simulink model "receiver_overall_reset"  (Simulink 7.5)
settings: Solver=FixedStepDiscrete  SolverMode=SingleTasking  StartTime=0.0  StopTime=(length(simin.signals.values)-1)/Fs  FixedStep=1  RelTol=1e-3
undefined symbols (not defined in the file): Fs
libraries: xbsIndex_r4 x962
(part 3 of 9)

== system receiver_overall_reset/Receiver/Sym-Chooser/7-15 ==
  in : Inport
  clk : Inport  Port=2
  0 : xbsIndex_r4/Constant  arith_type=Unsigned  const=a  n_bits=5  bin_pt=0  explicit_period=off  period=1  equ=P=C  opselect=C  inp2=PCIN>>17  opr=+  inp1=P  carry=CIN  dbl_ovrd=off  block_type=constant
      settings: block_version=12.1
  8 : xbsIndex_r4/Constant  arith_type=Unsigned  const=b  n_bits=5  bin_pt=0  explicit_period=off  period=1  equ=P=C  opselect=C  inp2=PCIN>>17  opr=+  inp1=P  carry=CIN  dbl_ovrd=off  block_type=constant
      settings: block_version=12.1
  Concat : xbsIndex_r4/Concat  num_inputs=2  dbl_ovrd=off  block_type=concat
      settings: block_version=12.1
  Corr0 : Subsystem
  Error0 : xbsIndex_r4/Constant  arith_type=Unsigned  const=16  n_bits=5  bin_pt=0  explicit_period=off  period=1  equ=P=C  opselect=C  inp2=PCIN>>17  opr=+  inp1=P  carry=CIN  dbl_ovrd=off  block_type=constant
      settings: block_version=12.1
  Error1 : xbsIndex_r4/Constant  arith_type=Unsigned  const=16  n_bits=5  bin_pt=0  explicit_period=off  period=1  equ=P=C  opselect=C  inp2=PCIN>>17  opr=+  inp1=P  carry=CIN  dbl_ovrd=off  block_type=constant
      settings: block_version=12.1
  Logical : xbsIndex_r4/Logical  logical_function=XOR  inputs=2  en=on  latency=1  precision=Full  arith_type=Unsigned  n_bits=16  bin_pt=0  align_bp=on  dbl_ovrd=off  block_type=logical
      settings: xl_area=[1 0 0 1 0 0 0]  block_version=12.1
  Mux : xbsIndex_r4/Mux  inputs=4  en=on  latency=1  precision=Full  arith_type=Unsigned  n_bits=16  bin_pt=14  quantization=Truncate  overflow=Wrap  dbl_ovrd=off  block_type=mux
      settings: xl_area=[5 5 0 10 0 0 0]  block_version=12.1
  Negate : xbsIndex_r4/Negate  precision=Full  arith_type="Signed  (2's comp)"  n_bits=16  bin_pt=14  quantization=Truncate  overflow=Wrap  en=off  latency=0  dbl_ovrd=off  block_type=negate
      settings: block_version=12.2
  Relational : xbsIndex_r4/Relational  mode=a>b  en=off  latency=0  dbl_ovrd=off  block_type=relational
      settings: xl_area=[4 1 0 7 0 0 0]  block_version=12.1
  Relational1 : xbsIndex_r4/Relational  mode=a<b  en=off  latency=0  dbl_ovrd=off  block_type=relational
      settings: xl_area=[4 1 0 7 0 0 0]  block_version=12.1
  Thresh : xbsIndex_r4/Constant  arith_type=Unsigned  const=thresh  n_bits=5  bin_pt=0  explicit_period=off  period=1  equ=P=C  opselect=C  inp2=PCIN>>17  opr=+  inp1=P  carry=CIN  dbl_ovrd=off  block_type=constant
      settings: block_version=12.1
  fnd : Outport
  value : Outport  Port=2
  wires:
  Corr0/1(Out1) -> Relational/1, Relational1/1
  Thresh/1 -> Relational/2, Negate/1
  in/1 -> Corr0/1(In1)
  Relational/1 -> Logical/1, Concat/1
  Relational1/1 -> Logical/2, Concat/2
  Logical/1 -> fnd/1
  Error0/1 -> Mux/2
  8/1 -> Mux/3
  Concat/1 -> Mux/1
  0/1 -> Mux/4
  Error1/1 -> Mux/5
  Mux/1 -> value/1
  Negate/1 -> Relational1/2
  clk/1 -> Mux/6, Logical/3

== system receiver_overall_reset/Receiver/Sym-Clk/Corr ==
  In : Inport
  AddSub : xbsIndex_r4/AddSub  mode=Subtraction  use_carryin=off  use_carryout=off  en=off  latency=0  precision=Full  arith_type=Unsigned  n_bits=16  bin_pt=14  quantization=Truncate  overflow=Wrap  dbl_ovrd=off  use_behavioral_HDL=off  hw_selection=Fabric  pipelined=off  block_type=addsub
      settings: xl_area=[4 0 0 6 0 0 0]  block_version=12.1
  Constant0 : xbsIndex_r4/Constant  arith_type=Unsigned  const=1618456172  n_bits=31  bin_pt=0  explicit_period=off  period=1/8  equ=P=C  opselect=C  inp2=PCIN>>17  opr=+  inp1=P  carry=CIN  dbl_ovrd=off  block_type=constant
      settings: block_version=12.1
  Constant1 : xbsIndex_r4/Constant  arith_type=Unsigned  const=31  n_bits=5  bin_pt=0  explicit_period=off  period=1/8  equ=P=C  opselect=C  inp2=PCIN>>17  opr=+  inp1=P  carry=CIN  dbl_ovrd=off  block_type=constant
      settings: block_version=12.1
  Delay_Line : Subsystem  mask{bits=31}
      mask prompts: bits "Number of Bits [2-40]"
      mask init:
      | % save_gcb = gcb
      | % nbits=bits+1
      | % old=find_system(save_gcb,...
      | %     'lookUnderMasks', 'all',...
      | %     'RegExp', 'On',...
      | %     'Name', 'DE\d+');
      | % 
      | %     for i=1:length(old)-1
      | %         delete_line(gcb, ['DE' int2str(i) '/1'], ['DE' int2str(i+1) '/1']);
      | %     end
      | %     for i=1:length(old)
      | %         delete_line(gcb, ['DE' int2str(i) '/2'], ['Concat/' int2str(length(old)-i+1)]);
      | %     end
      | %     delete_line(gcb, '1to2/2', ['Concat/', int2str(length(old)+1)]);
      | %     delete_line(gcb, ['DE' int2str(length(old)) '/1'], ['Terminator/1']);
      | %     for i=2:length(old)
      | %         delete_block(old{i});
      | %     end
      | % 
      | % pos = get_param([save_gcb '/DE1'], 'Position');
      | % width = pos(3)-pos(1);
      | % for i=3:nbits,
      | %     add_block([save_gcb '/DE1'],[save_gcb '/DE' int2str(i-1)],'position',[pos(1)+2*(i-2)*width, pos(2), pos(3)+2*(i-2)*width, pos(4)]);
      | %     add_line(save_gcb, ['DE' int2str(i-2) '/1'], ['DE' int2str(i-1) '/1'], 'autorouting', 'on');    
      | % end
      | % 
      | % posT = get_param([save_gcb '/Terminator'], 'Position');
      | % widthT = posT(3)-posT(1);
      | % heightT = posT(4)-posT(2);
      | % set_param([save_gcb '/Terminator'], 'Position', [pos(1)+2*(nbits-1)*width pos(2) pos(1)+2*(nbits-1)*width+widthT pos(2)+heightT]);
      | % 
      | % add_line(save_gcb, ['DE' int2str(nbits-1) '/1'], ['Terminator/1'], 'autorouting', 'on');
      | % 
      | % posC = get_param([save_gcb '/Concat'], 'Position');
      | % set_param([save_gcb '/Concat'], 'Position', [pos(1)+2*(nbits)*width posC(2) pos(1)+2*(nbits+1)*width posC(2)+2*(nbits-1)*width]);
      | % set_param([save_gcb '/Concat'], 'num_inputs', int2str(nbits));
      | % 
      | % add_line(save_gcb, '1to2/2', ['Concat/' int2str(nbits)], 'autorouting', 'on');
      | % for i=1:nbits-1,
      | %    add_line(save_gcb, ['DE' int2str(i) '/2'], ['Concat/' int2str(nbits-i)], 'autorouting', 'on');
      | % end
      mask StyleString: popup(2|3|4|5|6|7|8|9|10|11|12|13|14|15|16|17|18|19|20|21|22|23|24|25|26|27|28|29|30|31|32|33|34|35|36|37|38|39|40)
  Logical : xbsIndex_r4/Logical  logical_function=XNOR  inputs=2  en=off  latency=0  precision=User Defined  arith_type=Unsigned  n_bits=32  bin_pt=0  align_bp=on  dbl_ovrd=off  block_type=logical
      settings: xl_area=[31 0 0 31 0 0 0]  block_version=12.1
  count 1s : Subsystem
  x 2 : xbsIndex_r4/Shift  shift_dir=Left  shift_bits=1  en=off  latency=0  precision=Full  arith_type=Unsigned  n_bits=7  bin_pt=0  quantization=Truncate  overflow=Wrap  dbl_ovrd=off  block_type=shift
      settings: xl_area=[0 0 0 0 0 0 0]  block_version=12.1
  Out : Outport
  wires:
  Constant0/1 -> Logical/2
  Delay_Line/1(Out) -> Logical/1
  Logical/1 -> count 1s/1(in)
  Constant1/1 -> AddSub/2
  count 1s/1(out) -> x 2/1
  x 2/1 -> AddSub/1
  In/1 -> Delay_Line/1(In)
  AddSub/1 -> Out/1

== system receiver_overall_reset/Rule System/16bit Addresses + PANs/Adresses ==
  Dest Add Type : Inport
  Concat Symbols : Inport  Port=2
  Source Add Type : Inport  Port=3
  Source Add Settings : Inport  Port=4
  Dest Add Settings : Inport  Port=5
  1 : xbsIndex_r4/Constant  arith_type=Unsigned  const=2  n_bits=4  bin_pt=0  explicit_period=off  period=1  equ=P=C  opselect=C  inp2=PCIN>>17  opr=+  inp1=P  carry=CIN  dbl_ovrd=off  block_type=constant
      settings: block_version=12.2
  3 : xbsIndex_r4/Constant  arith_type=Unsigned  const=2  n_bits=4  bin_pt=0  explicit_period=off  period=1  equ=P=C  opselect=C  inp2=PCIN>>17  opr=+  inp1=P  carry=CIN  dbl_ovrd=off  block_type=constant
      settings: block_version=12.2
  Constant : xbsIndex_r4/Constant  arith_type=Unsigned  const=0  n_bits=16  bin_pt=0  explicit_period=off  period=1  equ=P=C  opselect=C  inp2=PCIN>>17  opr=+  inp1=P  carry=CIN  dbl_ovrd=off  block_type=constant
      settings: block_version=12.2
  Delay1 : xbsIndex_r4/Delay  en=off  latency=10  dbl_ovrd=off  reg_retiming=off  block_type=delay
      settings: block_version=12.2
  Delay2 : xbsIndex_r4/Delay  en=off  latency=18  dbl_ovrd=off  reg_retiming=off  block_type=delay
      settings: block_version=12.2
  Dest 16 upper Bound : xbsIndex_r4/Constant  arith_type=Unsigned  const=d16u  n_bits=16  bin_pt=0  explicit_period=off  period=1  equ=P=C  opselect=C  inp2=PCIN>>17  opr=+  inp1=P  carry=CIN  dbl_ovrd=off  block_type=constant
      settings: block_version=12.2
  Dest lower Bound : xbsIndex_r4/Constant  arith_type=Unsigned  const=d16l  n_bits=16  bin_pt=0  explicit_period=off  period=1  equ=P=C  opselect=C  inp2=PCIN>>17  opr=+  inp1=P  carry=CIN  dbl_ovrd=off  block_type=constant
      settings: block_version=12.2
  Logical : xbsIndex_r4/Logical  logical_function=AND  inputs=3  en=off  latency=0  precision=Full  arith_type=Unsigned  n_bits=16  bin_pt=0  align_bp=on  dbl_ovrd=off  block_type=logical
      settings: block_version=12.2
  Logical1 : xbsIndex_r4/Logical  logical_function=AND  inputs=3  en=off  latency=0  precision=Full  arith_type=Unsigned  n_bits=16  bin_pt=0  align_bp=on  dbl_ovrd=off  block_type=logical
      settings: block_version=12.2
  Logical2 : xbsIndex_r4/Logical  logical_function=OR  inputs=2  en=off  latency=0  precision=Full  arith_type=Unsigned  n_bits=16  bin_pt=0  align_bp=on  dbl_ovrd=off  block_type=logical
      settings: block_version=12.2
  Logical3 : xbsIndex_r4/Logical  logical_function=OR  inputs=2  en=off  latency=0  precision=Full  arith_type=Unsigned  n_bits=16  bin_pt=0  align_bp=on  dbl_ovrd=off  block_type=logical
      settings: block_version=12.2
  Logical4 : xbsIndex_r4/Logical  logical_function=OR  inputs=2  en=off  latency=0  precision=Full  arith_type=Unsigned  n_bits=16  bin_pt=0  align_bp=on  dbl_ovrd=off  block_type=logical
      settings: block_version=12.2
  Mux : xbsIndex_r4/Mux  inputs=2  en=off  latency=0  precision=Full  arith_type=Unsigned  n_bits=16  bin_pt=14  quantization=Truncate  overflow=Wrap  dbl_ovrd=off  block_type=mux
      settings: block_version=12.2
  Source 16 low Bound : xbsIndex_r4/Constant  arith_type=Unsigned  const=s16l  n_bits=16  bin_pt=0  explicit_period=off  period=1  equ=P=C  opselect=C  inp2=PCIN>>17  opr=+  inp1=P  carry=CIN  dbl_ovrd=off  block_type=constant
      settings: block_version=12.2
  Source 16 upper Bound : xbsIndex_r4/Constant  arith_type=Unsigned  const=s16u  n_bits=16  bin_pt=0  explicit_period=off  period=1  equ=P=C  opselect=C  inp2=PCIN>>17  opr=+  inp1=P  carry=CIN  dbl_ovrd=off  block_type=constant
      settings: block_version=12.2
  is{1..2,4..5} (4 alike) : xbsIndex_r4/Relational  mode=a>b  en=off  latency=0  dbl_ovrd=off  block_type=relational
      settings: block_version=12.2
  is16 : xbsIndex_r4/Relational  mode=a=b  en=off  latency=0  dbl_ovrd=off  block_type=relational
      settings: block_version=12.2
  is3 : xbsIndex_r4/Relational  mode=a=b  en=off  latency=0  dbl_ovrd=off  block_type=relational
      settings: block_version=12.2
  jam Dest Add : Outport
  jam Source Add : Outport  Port=2
  Source Type : Outport  Port=3
  Destination Type : Outport  Port=4
  Adress Value : Outport  Port=5
  wires:
  Concat Symbols/1 -> is4/1, is1/2, Mux/3, is5/1, is2/2
  3/1 -> is16/2
  is16/1 -> Delay1/1, Destination Type/1
  Delay1/1 -> Logical/1, Logical2/1
  Constant/1 -> Mux/2
  Logical2/1 -> Mux/1
  1/1 -> is3/2
  is3/1 -> Delay2/1, Source Type/1
  Delay2/1 -> Logical1/1, Logical2/2
  Dest Add Type/1 -> is16/1
  Logical/1 -> jam Dest Add/1
  Mux/1 -> Adress Value/1
  Logical1/1 -> jam Source Add/1
  Source Add Type/1 -> is3/1
  Source Add Settings/1 -> Logical1/3
  Dest Add Settings/1 -> Logical/3
  Dest lower Bound/1 -> is1/1
  Dest 16 upper Bound/1 -> is4/2
  is4/1 -> Logical3/2
  is1/1 -> Logical3/1
  Logical3/1 -> Logical/2
  Source 16 low Bound/1 -> is2/1
  Source 16 upper Bound/1 -> is5/2
  is5/1 -> Logical4/2
  is2/1 -> Logical4/1
  Logical4/1 -> Logical1/2

== system receiver_overall_reset/Rule System/16bit Addresses + PANs/PANs ==
  Concat Symbols : Inport
  Dest PanType : Inport  Port=2
  Source PanType : Inport  Port=3
  Dest PAN Settings : Inport  Port=4
  Source Pan Settings : Inport  Port=5
  Constant : xbsIndex_r4/Constant  arith_type=Unsigned  const=0  n_bits=16  bin_pt=0  explicit_period=off  period=1  equ=P=C  opselect=C  inp2=PCIN>>17  opr=+  inp1=P  carry=CIN  dbl_ovrd=off  block_type=constant
      settings: block_version=12.2
  Delay1 : xbsIndex_r4/Delay  en=off  latency=6  dbl_ovrd=off  reg_retiming=off  block_type=delay
      settings: block_version=12.2
  Delay2 : xbsIndex_r4/Delay  en=off  latency=14  dbl_ovrd=off  reg_retiming=off  block_type=delay
      settings: block_version=12.2
  Dest PAN lower bound : xbsIndex_r4/Constant  arith_type=Unsigned  const=dpl  n_bits=16  bin_pt=0  explicit_period=off  period=1  equ=P=C  opselect=C  inp2=PCIN>>17  opr=+  inp1=P  carry=CIN  dbl_ovrd=off  block_type=constant
      settings: block_version=12.2
  Dest PAN upper bound : xbsIndex_r4/Constant  arith_type=Unsigned  const=dpu  n_bits=16  bin_pt=0  explicit_period=off  period=1  equ=P=C  opselect=C  inp2=PCIN>>17  opr=+  inp1=P  carry=CIN  dbl_ovrd=off  block_type=constant
      settings: block_version=12.2
  Logical : xbsIndex_r4/Logical  logical_function=AND  inputs=3  en=off  latency=0  precision=Full  arith_type=Unsigned  n_bits=16  bin_pt=0  align_bp=on  dbl_ovrd=off  block_type=logical
      settings: block_version=12.2
  Logical1 : xbsIndex_r4/Logical  logical_function=AND  inputs=3  en=off  latency=0  precision=Full  arith_type=Unsigned  n_bits=16  bin_pt=0  align_bp=on  dbl_ovrd=off  block_type=logical
      settings: block_version=12.2
  Logical2 : xbsIndex_r4/Logical  logical_function=OR  inputs=2  en=off  latency=0  precision=Full  arith_type=Unsigned  n_bits=16  bin_pt=0  align_bp=on  dbl_ovrd=off  block_type=logical
      settings: block_version=12.2
  Logical3 : xbsIndex_r4/Logical  logical_function=OR  inputs=2  en=off  latency=0  precision=Full  arith_type=Unsigned  n_bits=16  bin_pt=0  align_bp=on  dbl_ovrd=off  block_type=logical
      settings: block_version=12.2
  Logical4 : xbsIndex_r4/Logical  logical_function=OR  inputs=2  en=off  latency=0  precision=Full  arith_type=Unsigned  n_bits=16  bin_pt=0  align_bp=on  dbl_ovrd=off  block_type=logical
      settings: block_version=12.2
  Mux : xbsIndex_r4/Mux  inputs=2  en=off  latency=0  precision=Full  arith_type=Unsigned  n_bits=16  bin_pt=14  quantization=Truncate  overflow=Wrap  dbl_ovrd=off  block_type=mux
      settings: block_version=12.2
  Source PAN lower bound : xbsIndex_r4/Constant  arith_type=Unsigned  const=spl  n_bits=16  bin_pt=0  explicit_period=off  period=1  equ=P=C  opselect=C  inp2=PCIN>>17  opr=+  inp1=P  carry=CIN  dbl_ovrd=off  block_type=constant
      settings: block_version=12.2
  Source PAN upper bound : xbsIndex_r4/Constant  arith_type=Unsigned  const=spu  n_bits=16  bin_pt=0  explicit_period=off  period=1  equ=P=C  opselect=C  inp2=PCIN>>17  opr=+  inp1=P  carry=CIN  dbl_ovrd=off  block_type=constant
      settings: block_version=12.2
  is{1..4} (4 alike) : xbsIndex_r4/Relational  mode=a>b  en=off  latency=0  dbl_ovrd=off  block_type=relational
      settings: block_version=12.2
  jam Dest PAN : Outport
  PAN Value : Outport  Port=2
  jam Source PAN : Outport  Port=3
  wires:
  Concat Symbols/1 -> is3/1, is1/2, Mux/3, is4/1, is2/2
  Dest PanType/1 -> Delay1/1
  Delay1/1 -> Logical/1, Logical2/1
  Constant/1 -> Mux/2
  Logical2/1 -> Mux/1
  Source PanType/1 -> Delay2/1
  Delay2/1 -> Logical1/1, Logical2/2
  Logical/1 -> jam Dest PAN/1
  Mux/1 -> PAN Value/1
  Logical1/1 -> jam Source PAN/1
  Dest PAN Settings/1 -> Logical/3
  Source Pan Settings/1 -> Logical1/3
  Dest PAN lower bound/1 -> is1/1
  Dest PAN upper bound/1 -> is3/2
  is3/1 -> Logical3/2
  is1/1 -> Logical3/1
  Logical3/1 -> Logical/2
  Source PAN lower bound/1 -> is2/1
  Source PAN upper bound/1 -> is4/2
  is4/1 -> Logical4/2
  is2/1 -> Logical4/1
  Logical4/1 -> Logical1/2

== system receiver_overall_reset/Rule System/64bit Addresses/Subsystem ==
  Add Left : Inport
  Add Rigth : Inport  Port=2
  Low Left : Inport  Port=3
  Low Right : Inport  Port=4
  Up Left : Inport  Port=5
  Up Rigth : Inport  Port=6
  Logical1 : xbsIndex_r4/Logical  logical_function=OR  inputs=2  en=off  latency=0  precision=Full  arith_type=Unsigned  n_bits=16  bin_pt=0  align_bp=on  dbl_ovrd=off  block_type=logical
      settings: block_version=12.2
  Logical3 : xbsIndex_r4/Logical  logical_function=OR  inputs=2  en=off  latency=0  precision=Full  arith_type=Unsigned  n_bits=16  bin_pt=0  align_bp=on  dbl_ovrd=off  block_type=logical
      settings: block_version=12.2
  Logical5 : xbsIndex_r4/Logical  logical_function=OR  inputs=2  en=off  latency=0  precision=Full  arith_type=Unsigned  n_bits=16  bin_pt=0  align_bp=on  dbl_ovrd=off  block_type=logical
      settings: block_version=12.2
  Relational : xbsIndex_r4/Relational  mode=a<b  en=off  latency=0  dbl_ovrd=off  block_type=relational
      settings: block_version=12.2
  Relational1 : xbsIndex_r4/Relational  mode=a=b  en=off  latency=0  dbl_ovrd=off  block_type=relational
      settings: block_version=12.2
  Relational2 : xbsIndex_r4/Relational  mode=a<b  en=off  latency=0  dbl_ovrd=off  block_type=relational
      settings: block_version=12.2
  Relational3 : xbsIndex_r4/Relational  mode=a>b  en=off  latency=0  dbl_ovrd=off  block_type=relational
      settings: block_version=12.2
  Relational4 : xbsIndex_r4/Relational  mode=a=b  en=off  latency=0  dbl_ovrd=off  block_type=relational
      settings: block_version=12.2
  Relational5 : xbsIndex_r4/Relational  mode=a>b  en=off  latency=0  dbl_ovrd=off  block_type=relational
      settings: block_version=12.2
  and : xbsIndex_r4/Logical  logical_function=AND  inputs=2  en=off  latency=0  precision=Full  arith_type=Unsigned  n_bits=16  bin_pt=0  align_bp=on  dbl_ovrd=off  block_type=logical
      settings: block_version=12.2
  and1 : xbsIndex_r4/Logical  logical_function=AND  inputs=2  en=off  latency=0  precision=Full  arith_type=Unsigned  n_bits=16  bin_pt=0  align_bp=on  dbl_ovrd=off  block_type=logical
      settings: block_version=12.2
  Dest 64b Jam : Outport
  wires:
  Add Left/1 -> Relational/1, Relational1/1, Relational3/1, Relational4/1
  Low Left/1 -> Relational/2, Relational1/2
  Relational/1 -> Logical1/1
  Relational2/1 -> and/2
  Relational1/1 -> and/1
  and/1 -> Logical1/2
  Add Rigth/1 -> Relational2/1, Relational5/1
  Low Right/1 -> Relational2/2
  Relational3/1 -> Logical3/1
  Relational5/1 -> and1/2
  Relational4/1 -> and1/1
  and1/1 -> Logical3/2
  Up Left/1 -> Relational3/2, Relational4/2
  Up Rigth/1 -> Relational5/2
  Logical1/1 -> Logical5/1
  Logical3/1 -> Logical5/2
  Logical5/1 -> Dest 64b Jam/1

== system receiver_overall_reset/Rule System/64bit Addresses/Subsystem1 ==
  Add Left : Inport
  Add Rigth : Inport  Port=2
  Low Left : Inport  Port=3
  Low Right : Inport  Port=4
  Up Left : Inport  Port=5
  Up Rigth : Inport  Port=6
  Logical1 : xbsIndex_r4/Logical  logical_function=OR  inputs=2  en=off  latency=0  precision=Full  arith_type=Unsigned  n_bits=16  bin_pt=0  align_bp=on  dbl_ovrd=off  block_type=logical
      settings: block_version=12.2
  Logical2 : xbsIndex_r4/Logical  logical_function=AND  inputs=2  en=off  latency=0  precision=Full  arith_type=Unsigned  n_bits=16  bin_pt=0  align_bp=on  dbl_ovrd=off  block_type=logical
      settings: block_version=12.2
  Logical3 : xbsIndex_r4/Logical  logical_function=OR  inputs=2  en=off  latency=0  precision=Full  arith_type=Unsigned  n_bits=16  bin_pt=0  align_bp=on  dbl_ovrd=off  block_type=logical
      settings: block_version=12.2
  Logical4 : xbsIndex_r4/Logical  logical_function=AND  inputs=2  en=off  latency=0  precision=Full  arith_type=Unsigned  n_bits=16  bin_pt=0  align_bp=on  dbl_ovrd=off  block_type=logical
      settings: block_version=12.2
  Logical5 : xbsIndex_r4/Logical  logical_function=OR  inputs=2  en=off  latency=0  precision=Full  arith_type=Unsigned  n_bits=16  bin_pt=0  align_bp=on  dbl_ovrd=off  block_type=logical
      settings: block_version=12.2
  Relational : xbsIndex_r4/Relational  mode=a<b  en=off  latency=0  dbl_ovrd=off  block_type=relational
      settings: block_version=12.2
  Relational1 : xbsIndex_r4/Relational  mode=a=b  en=off  latency=0  dbl_ovrd=off  block_type=relational
      settings: block_version=12.2
  Relational2 : xbsIndex_r4/Relational  mode=a<b  en=off  latency=0  dbl_ovrd=off  block_type=relational
      settings: block_version=12.2
  Relational3 : xbsIndex_r4/Relational  mode=a>b  en=off  latency=0  dbl_ovrd=off  block_type=relational
      settings: block_version=12.2
  Relational4 : xbsIndex_r4/Relational  mode=a=b  en=off  latency=0  dbl_ovrd=off  block_type=relational
      settings: block_version=12.2
  Relational5 : xbsIndex_r4/Relational  mode=a>b  en=off  latency=0  dbl_ovrd=off  block_type=relational
      settings: block_version=12.2
  Out1 : Outport
  wires:
  Add Left/1 -> Relational/1, Relational1/1, Relational3/1, Relational4/1
  Low Left/1 -> Relational/2, Relational1/2
  Relational/1 -> Logical1/1  "low l grt"
  Relational2/1 -> Logical2/2  "low r grt"
  Relational1/1 -> Logical2/1  "low equal"
  Logical2/1 -> Logical1/2
  Add Rigth/1 -> Relational2/1, Relational5/1
  Low Right/1 -> Relational2/2
  Relational3/1 -> Logical3/1  "up l grt"
  Relational5/1 -> Logical4/2  "up r grt"
  Relational4/1 -> Logical4/1  "up equal"
  Logical4/1 -> Logical3/2
  Up Left/1 -> Relational3/2, Relational4/2
  Up Rigth/1 -> Relational5/2
  Logical1/1 -> Logical5/1
  Logical3/1 -> Logical5/2
  Logical5/1 -> Out1/1

== system receiver_overall_reset/Rule System/Header Analyser/type analyser ==
  choose_type : Inport
  type_header_bits : Inport  Port=2
  0 : xbsIndex_r4/Constant  arith_type=Unsigned  const=0  n_bits=4  bin_pt=0  explicit_period=off  period=1  equ=P=C  opselect=C  inp2=PCIN>>17  opr=+  inp1=P  carry=CIN  dbl_ovrd=off  block_type=constant
      settings: block_version=12.2
  1 : xbsIndex_r4/Constant  arith_type=Boolean  const=0  n_bits=4  bin_pt=0  explicit_period=off  period=1  equ=P=C  opselect=C  inp2=PCIN>>17  opr=+  inp1=P  carry=CIN  dbl_ovrd=off  block_type=constant
      settings: block_version=12.2
  4 : xbsIndex_r4/Constant  arith_type=Unsigned  const=3  n_bits=4  bin_pt=0  explicit_period=off  period=1  equ=P=C  opselect=C  inp2=PCIN>>17  opr=+  inp1=P  carry=CIN  dbl_ovrd=off  block_type=constant
      settings: block_version=12.2
  Logical : xbsIndex_r4/Logical  logical_function=OR  inputs=2  en=off  latency=0  precision=Full  arith_type=Unsigned  n_bits=16  bin_pt=0  align_bp=on  dbl_ovrd=off  block_type=logical
      settings: block_version=12.2
  Mux3 : xbsIndex_r4/Mux  inputs=4  en=off  latency=0  precision=Full  arith_type=Unsigned  n_bits=16  bin_pt=14  quantization=Truncate  overflow=Wrap  dbl_ovrd=off  block_type=mux
      settings: block_version=12.2
  isBeacon : xbsIndex_r4/Relational  mode=a=b  en=off  latency=0  dbl_ovrd=off  block_type=relational
      settings: block_version=12.2
  isMAC : xbsIndex_r4/Relational  mode=a=b  en=off  latency=0  dbl_ovrd=off  block_type=relational
      settings: block_version=12.2
  jam_type : Outport
  wires:
  0/1 -> isBeacon/2
  4/1 -> isMAC/2
  isBeacon/1 -> Logical/1, Mux3/4
  type_header_bits/1 -> isBeacon/1, isMAC/1
  choose_type/1 -> Mux3/1
  Mux3/1 -> jam_type/1
  isMAC/1 -> Mux3/3, Logical/2
  Logical/1 -> Mux3/5
  1/1 -> Mux3/2

== system receiver_overall_reset/Receiver/FM demod/CORDIC ATAN/CORDIC Fine Angle PE ==
  note: The fine angle rotation operation is performed iteratively in stages (0..stages-1).
      | The i-th PE rotates its input vector by an angle +/- atan(1/2^i), driving its input y coordinate towards zero.
  x : Inport  OutDataType=sfix(16)  OutScaling=2^0
  y : Inport  Port=2  OutDataType=sfix(16)  OutScaling=2^0
  z : Inport  Port=3  OutDataType=sfix(16)  OutScaling=2^0
  CORDIC PE1 : Subsystem  mask(CORDIC iteration PE){ii=0, pe_nbits=pe_nbits, pe_binpt=pe_binpt, epsilon_k_fcn=atan, epsilon_k=, pipeline=pipeline(1,1)}
      mask prompts: ii "Iteration Index ii"; pe_nbits "Number of X,Y,Z Bits"; pe_binpt "X,Y,Z Binary Point Position"; epsilon_k_fcn "Epsilon_k Function"; pipeline "Pipeline Latency"
      mask init:
      | [bg,fg] = xlcmap('XBlock',0);
      | iPos = get_param(gcb,'Position');
      | iWidth=iPos(3)-iPos(1); iHeight=iPos(4)-iPos(2);
      | iCx=iWidth/2;
      | iCy=iHeight/2;
      | [logoX, logoY] = xlogo(iPos);
      | 
      | set_param(gcb, 'LinkStatus', 'none');
      | switch epsilon_k_fcn
      |   case 1
      |     epsilon_k = atan(1/2^ii);
      |   case 2
      |     epsilon_k = atanh(1/2^ii);
      | end
      mask StyleString: edit,edit,edit,popup(atan|atanh),edit,edit
      mask Display:
      | patch([0 iWidth iWidth 0],[0 0 iHeight iHeight] , bg);
      | patch(logoX,logoY , fg);
      | port_label('input',1,'x');
      | port_label('input',2,'y');
      | port_label('input',3,'z');
      | port_label('output',1,'X');
      | port_label('output',2,'Y');
      | port_label('output',3,'Z');
      | plot([0 0 iWidth iWidth 0], [0 iHeight iHeight 0 0]);
  CORDIC PE2 : Subsystem  mask(CORDIC iteration PE){ii=1, pe_nbits=pe_nbits, pe_binpt=pe_binpt, epsilon_k_fcn=atan, epsilon_k=, pipeline=pipeline(1,2)}
      mask prompts: ii "Iteration Index ii"; pe_nbits "Number of X,Y,Z Bits"; pe_binpt "X,Y,Z Binary Point Position"; epsilon_k_fcn "Epsilon_k Function"; pipeline "Pipeline Latency"
      mask init: same as receiver_overall_reset/Receiver/FM demod/CORDIC ATAN/CORDIC Fine Angle PE/CORDIC PE1
      mask StyleString: edit,edit,edit,popup(atan|atanh),edit,edit
      mask Display:
      | patch([0 iWidth iWidth 0],[0 0 iHeight iHeight] , bg);
      | patch(logoX,logoY , fg);
      | port_label('input',1,'x');
      | port_label('input',2,'y');
      | port_label('input',3,'z');
      | port_label('output',1,'X');
      | port_label('output',2,'Y');
      | port_label('output',3,'Z');
      | plot([0 0 iWidth iWidth 0], [0 iHeight iHeight 0 0]);
  CORDIC PE3 : Subsystem  mask(CORDIC iteration PE){ii=2, pe_nbits=pe_nbits, pe_binpt=pe_binpt, epsilon_k_fcn=atan, epsilon_k=, pipeline=pipeline(1,3)}
      mask prompts: ii "Iteration Index ii"; pe_nbits "Number of X,Y,Z Bits"; pe_binpt "X,Y,Z Binary Point Position"; epsilon_k_fcn "Epsilon_k Function"; pipeline "Pipeline Latency"
      mask init: same as receiver_overall_reset/Receiver/FM demod/CORDIC ATAN/CORDIC Fine Angle PE/CORDIC PE1
      mask StyleString: edit,edit,edit,popup(atan|atanh),edit,edit
      mask Display:
      | patch([0 iWidth iWidth 0],[0 0 iHeight iHeight] , bg);
      | patch(logoX,logoY , fg);
      | port_label('input',1,'x');
      | port_label('input',2,'y');
      | port_label('input',3,'z');
      | port_label('output',1,'X');
      | port_label('output',2,'Y');
      | port_label('output',3,'Z');
      | plot([0 0 iWidth iWidth 0], [0 iHeight iHeight 0 0]);
  CORDIC PE4 : Subsystem  mask(CORDIC iteration PE){ii=3, pe_nbits=pe_nbits, pe_binpt=pe_binpt, epsilon_k_fcn=atan, epsilon_k=, pipeline=pipeline(1,4)}
      mask prompts: ii "Iteration Index ii"; pe_nbits "Number of X,Y,Z Bits"; pe_binpt "X,Y,Z Binary Point Position"; epsilon_k_fcn "Epsilon_k Function"; pipeline "Pipeline Latency"
      mask init: same as receiver_overall_reset/Receiver/FM demod/CORDIC ATAN/CORDIC Fine Angle PE/CORDIC PE1
      mask StyleString: edit,edit,edit,popup(atan|atanh),edit,edit
      mask Display:
      | patch([0 iWidth iWidth 0],[0 0 iHeight iHeight] , bg);
      | patch(logoX,logoY , fg);
      | port_label('input',1,'x');
      | port_label('input',2,'y');
      | port_label('input',3,'z');
      | port_label('output',1,'X');
      | port_label('output',2,'Y');
      | port_label('output',3,'Z');
      | plot([0 0 iWidth iWidth 0], [0 iHeight iHeight 0 0]);
  CORDIC PE5 : Subsystem  mask(CORDIC iteration PE){ii=4, pe_nbits=pe_nbits, pe_binpt=pe_binpt, epsilon_k_fcn=atan, epsilon_k=, pipeline=pipeline(1,5)}
      mask prompts: ii "Iteration Index ii"; pe_nbits "Number of X,Y,Z Bits"; pe_binpt "X,Y,Z Binary Point Position"; epsilon_k_fcn "Epsilon_k Function"; pipeline "Pipeline Latency"
      mask init: same as receiver_overall_reset/Receiver/FM demod/CORDIC ATAN/CORDIC Fine Angle PE/CORDIC PE1
      mask StyleString: edit,edit,edit,popup(atan|atanh),edit,edit
      mask Display:
      | patch([0 iWidth iWidth 0],[0 0 iHeight iHeight] , bg);
      | patch(logoX,logoY , fg);
      | port_label('input',1,'x');
      | port_label('input',2,'y');
      | port_label('input',3,'z');
      | port_label('output',1,'X');
      | port_label('output',2,'Y');
      | port_label('output',3,'Z');
      | plot([0 0 iWidth iWidth 0], [0 iHeight iHeight 0 0]);
  Terminator : Terminator
  X : Outport  OutDataType=sfix(16)  OutScaling=2^0
  Z : Outport  Port=2  OutDataType=sfix(16)  OutScaling=2^0
  wires:
  CORDIC PE1/1(X) -> CORDIC PE2/1(x)
  CORDIC PE1/2(Y) -> CORDIC PE2/2(y)
  CORDIC PE1/3(Z) -> CORDIC PE2/3(z)
  CORDIC PE2/1(X) -> CORDIC PE3/1(x)
  CORDIC PE2/2(Y) -> CORDIC PE3/2(y)
  CORDIC PE2/3(Z) -> CORDIC PE3/3(z)
  CORDIC PE3/1(X) -> CORDIC PE4/1(x)
  CORDIC PE3/2(Y) -> CORDIC PE4/2(y)
  CORDIC PE3/3(Z) -> CORDIC PE4/3(z)
  CORDIC PE4/1(X) -> CORDIC PE5/1(x)
  CORDIC PE4/2(Y) -> CORDIC PE5/2(y)
  CORDIC PE4/3(Z) -> CORDIC PE5/3(z)
  x/1 -> CORDIC PE1/1(x)
  y/1 -> CORDIC PE1/2(y)
  z/1 -> CORDIC PE1/3(z)
  CORDIC PE5/1(X) -> X/1
  CORDIC PE5/2(Y) -> Terminator/1
  CORDIC PE5/3(Z) -> Z/1

== system receiver_overall_reset/Receiver/FM demod/CORDIC ATAN/Quadrant Correct ==
  note: The  CORDIC algorithm coverges for angles between  -pi/2 to +pi/2. The Quadrant Correct subsystem reflects
      | the angle back to the 2nd and 3rd quadrant from the 1st and 4th quadarnt if reflection was applied during the
      | quadarnt map stage. Reflection is applied by subtracting the output angle by pi if the original vector was in the
      | 2nd quadrant and -p if it was in the 3rd quadrant.
  Z IN : Inport  OutDataType=sfix(16)  OutScaling=2^0
  PI_ addsub : Inport  Port=2  OutDataType=sfix(16)  OutScaling=2^0
  Z MUX SEL : Inport  Port=3  OutDataType=sfix(16)  OutScaling=2^0
  +PI : xbsIndex_r4/Constant  arith_type=Signed (2's comp)  const=pi  n_bits=pe_nbits  bin_pt=pe_binpt  explicit_period=off  period=1  equ=P=C  opselect=C  inp2=PCIN>>17  opr=+  inp1=P  carry=CIN  dbl_ovrd=off  block_type=constant
      settings: block_version=VER_STRING_GOES_HERE
  -PI : xbsIndex_r4/Constant  arith_type=Signed (2's comp)  const=-pi  n_bits=pe_nbits  bin_pt=pe_binpt  explicit_period=off  period=1  equ=P=C  opselect=C  inp2=PCIN>>17  opr=+  inp1=P  carry=CIN  dbl_ovrd=off  block_type=constant
      settings: block_version=VER_STRING_GOES_HERE
  AddSub : xbsIndex_r4/AddSub  mode=Subtraction  use_carryin=off  use_carryout=off  en=off  latency=0  precision=User Defined  arith_type="Signed  (2's comp)"  n_bits=pe_nbits  bin_pt=pe_binpt  quantization=Truncate  overflow=Wrap  dbl_ovrd=off  use_behavioral_HDL=on  hw_selection=Fabric  pipelined=off  use_rpm=off  block_type=addsub
      settings: xl_area=[17 0 0 33 0 0 0]  block_version=VER_STRING_GOES_HERE
  Convert : xbsIndex_r4/Convert  arith_type=Boolean  n_bits=8  bin_pt=6  quantization=Truncate  overflow=Wrap  en=off  latency=0  dbl_ovrd=off  pipeline=off  block_type=convert
      settings: infoedit=The input is presented at the output after quantization and overflow effects.<P><P>Hardware notes: Additional hardware is used when rounding or saturation is selected and output width is less than the input width.  xl_area=[0 0 0 0 0 0 0]  block_version=VER_STRING_GOES_HERE
  Mux : xbsIndex_r4/Mux  inputs=2  en=off  latency=1  precision=Full  arith_type="Signed  (2's comp)"  n_bits=8  bin_pt=2  quantization=Truncate  overflow=Wrap  dbl_ovrd=off  block_type=mux
      settings: xl_area=[17 33 0 33 0 0 0]  infoedit=Binary points are aligned automatically.<P><P>Hardware notes: A multiplexer using tristate buffers requires fewer lookup tables but is slower.  block_version=VER_STRING_GOES_HERE
  Mux1 : xbsIndex_r4/Mux  inputs=2  en=off  latency=0  precision=Full  arith_type="Signed  (2's comp)"  n_bits=8  bin_pt=2  quantization=Truncate  overflow=Wrap  dbl_ovrd=off  block_type=mux
      settings: xl_area=[17 0 0 33 0 0 0]  infoedit=Binary points are aligned automatically.<P><P>Hardware notes: A multiplexer using tristate buffers requires fewer lookup tables but is slower.  block_version=VER_STRING_GOES_HERE
  Z : Outport  OutDataType=sfix(16)  OutScaling=2^0
  wires:
  PI_ addsub/1 -> Convert/1
  Z MUX SEL/1 -> Mux/1
  AddSub/1 -> Mux/3
  Mux/1 -> Z/1
  Z IN/1 -> AddSub/2, Mux/2
  Convert/1 -> Mux1/1
  Mux1/1 -> AddSub/1
  +PI/1 -> Mux1/2
  -PI/1 -> Mux1/3

== system receiver_overall_reset/Receiver/FM demod/CORDIC ATAN/Quadrant Map ==
  note: The  CORDIC algorithm converges for angles between  -pi/2 to +pi/2. The Quadrant Map subsystem always maps the
      | absolute value for x-axis. This reflects the input vector from the 2nd and 3rd quadrant to the 1st and 4th quadrant, resp.
  x : Inport  OutDataType=sfix(16)  OutScaling=2^0
  y : Inport  Port=2  OutDataType=sfix(16)  OutScaling=2^0
  Delay3 : xbsIndex_r4/Delay  en=off  latency=2  dbl_ovrd=off  reg_retiming=off  block_type=delay
      settings: infoedit="Delay line having  configurable length.<P><P>Hardware notes: A delay line is a chain, each link of which is an SRL16 followed by a flip-flop. If register retiming is enabled, the delay line is a chain of flip-flops."  xl_area=[17 33 0 33 0 0 0]  block_version=VER_STRING_GOES_HERE
  Delay4 : xbsIndex_r4/Delay  en=off  latency=1  dbl_ovrd=off  reg_retiming=off  block_type=delay
      settings: infoedit="Delay line having  configurable length.<P><P>Hardware notes: A delay line is a chain, each link of which is an SRL16 followed by a flip-flop. If register retiming is enabled, the delay line is a chain of flip-flops."  xl_area=[17 33 0 0 0 0 0]  block_version=VER_STRING_GOES_HERE
  Mux : xbsIndex_r4/Mux  inputs=2  en=off  latency=1  precision=User Defined  arith_type="Signed  (2's comp)"  n_bits=pe_nbits  bin_pt=pe_binpt  quantization=Truncate  overflow=Wrap  dbl_ovrd=off  block_type=mux
      settings: xl_area=[17 33 0 33 0 0 0]  infoedit=Binary points are aligned automatically.<P><P>Hardware notes: A multiplexer using tristate buffers requires fewer lookup tables but is slower.  block_version=VER_STRING_GOES_HERE
  Negate1 : xbsIndex_r4/Negate  precision=User Defined  arith_type="Signed  (2's comp)"  n_bits=pe_nbits  bin_pt=pe_binpt  quantization=Truncate  overflow=Wrap  en=off  latency=0  dbl_ovrd=off  block_type=negate
      settings: xl_area=[17 0 0 33 0 0 0]  block_version=VER_STRING_GOES_HERE
  sgn(x) : xbsIndex_r4/Slice  nbits=1  boolean_output=off  mode=Upper Bit Location + Width  bit1=0  base1=MSB of Input  bit0=0  base0=LSB of Input  dbl_ovrd=off  block_type=slice
      settings: infoedit="Extracts a given range of bits from each input sample and presents it at the output.  The output type is ordinarily unsigned with binary point at zero, but can be Boolean when the slice is one bit wide.<P><P>Hardware notes: In hardware this block costs nothing."  block_version=VER_STRING_GOES_HERE
  sgn(y) : xbsIndex_r4/Slice  nbits=1  boolean_output=off  mode=Upper Bit Location + Width  bit1=0  base1=MSB of Input  bit0=0  base0=LSB of Input  dbl_ovrd=off  block_type=slice
      settings: infoedit="Extracts a given range of bits from each input sample and presents it at the output.  The output type is ordinarily unsigned with binary point at zero, but can be Boolean when the slice is one bit wide.<P><P>Hardware notes: In hardware this block costs nothing."  block_version=VER_STRING_GOES_HERE
  X : Outport  OutDataType=sfix(16)  OutScaling=2^0
  Y : Outport  Port=2  OutDataType=sfix(16)  OutScaling=2^0
  sign(y) : Outport  Port=3  OutDataType=sfix(16)  OutScaling=2^0
  sign(x) : Outport  Port=4  OutDataType=sfix(16)  OutScaling=2^0
  wires:
  Delay4/1 -> Mux/2, Negate1/1, sgn(x)/1
  sgn(y)/1 -> sign(y)/1
  sgn(x)/1 -> sign(x)/1, Mux/1
  x/1 -> Delay4/1
  y/1 -> Delay3/1
  Mux/1 -> X/1
  Negate1/1 -> Mux/3
  Delay3/1 -> sgn(y)/1, Y/1

== system receiver_overall_reset/Receiver/Sym-Chooser/0-8/Corr0 ==
  In : Inport
  AddSub : xbsIndex_r4/AddSub  mode=Subtraction  use_carryin=off  use_carryout=off  en=off  latency=0  precision=Full  arith_type=Unsigned  n_bits=16  bin_pt=14  quantization=Truncate  overflow=Wrap  dbl_ovrd=off  use_behavioral_HDL=off  hw_selection=Fabric  pipelined=off  block_type=addsub
      settings: xl_area=[4 0 0 6 0 0 0]  block_version=12.1
  Constant0 : xbsIndex_r4/Constant  arith_type=Unsigned  const=chip_a  n_bits=31  bin_pt=0  explicit_period=off  period=1/8  equ=P=C  opselect=C  inp2=PCIN>>17  opr=+  inp1=P  carry=CIN  dbl_ovrd=off  block_type=constant
      settings: block_version=12.1
  Constant1 : xbsIndex_r4/Constant  arith_type=Unsigned  const=31  n_bits=5  bin_pt=0  explicit_period=off  period=1/8  equ=P=C  opselect=C  inp2=PCIN>>17  opr=+  inp1=P  carry=CIN  dbl_ovrd=off  block_type=constant
      settings: block_version=12.1
  Corr : Subsystem
  Delay_Line : Subsystem  mask{bits=31}
      mask prompts: bits "Number of Bits [2-40]"
      mask init: same as receiver_overall_reset/Receiver/Sym-Clk/Corr/Delay_Line
      mask StyleString: popup(2|3|4|5|6|7|8|9|10|11|12|13|14|15|16|17|18|19|20|21|22|23|24|25|26|27|28|29|30|31|32|33|34|35|36|37|38|39|40)
  Logical : xbsIndex_r4/Logical  logical_function=XNOR  inputs=2  en=off  latency=0  precision=User Defined  arith_type=Unsigned  n_bits=32  bin_pt=0  align_bp=on  dbl_ovrd=off  block_type=logical
      settings: xl_area=[31 0 0 31 0 0 0]  block_version=12.1
  Shift : xbsIndex_r4/Shift  shift_dir=Left  shift_bits=1  en=off  latency=0  precision=Full  arith_type=Unsigned  n_bits=7  bin_pt=0  quantization=Truncate  overflow=Wrap  dbl_ovrd=off  block_type=shift
      settings: xl_area=[0 0 0 0 0 0 0]  block_version=12.1
  Out : Outport
  wires:
  Constant0/1 -> Logical/2
  Delay_Line/1(Out2) -> Logical/1
  Logical/1 -> Corr/1(In1)
  Constant1/1 -> AddSub/2
  Corr/1(Out2) -> Shift/1
  Shift/1 -> AddSub/1
  In/1 -> Delay_Line/1(In1)
  AddSub/1 -> Out/1

== system receiver_overall_reset/Receiver/Sym-Chooser/1-9/Corr0 ==
  In1 : Inport
  AddSub : xbsIndex_r4/AddSub  mode=Subtraction  use_carryin=off  use_carryout=off  en=off  latency=0  precision=Full  arith_type=Unsigned  n_bits=16  bin_pt=14  quantization=Truncate  overflow=Wrap  dbl_ovrd=off  use_behavioral_HDL=off  hw_selection=Fabric  pipelined=off  block_type=addsub
      settings: xl_area=[4 0 0 6 0 0 0]  block_version=12.1
  Constant0 : xbsIndex_r4/Constant  arith_type=Unsigned  const=chip_a  n_bits=31  bin_pt=0  explicit_period=off  period=1/8  equ=P=C  opselect=C  inp2=PCIN>>17  opr=+  inp1=P  carry=CIN  dbl_ovrd=off  block_type=constant
      settings: block_version=12.1
  Constant1 : xbsIndex_r4/Constant  arith_type=Unsigned  const=31  n_bits=5  bin_pt=0  explicit_period=off  period=1/8  equ=P=C  opselect=C  inp2=PCIN>>17  opr=+  inp1=P  carry=CIN  dbl_ovrd=off  block_type=constant
      settings: block_version=12.1
  Corr : Subsystem
  Delay_Line : Subsystem  mask{bits=31}
      mask prompts: bits "Number of Bits [2-40]"
      mask init: same as receiver_overall_reset/Receiver/Sym-Clk/Corr/Delay_Line
      mask StyleString: popup(2|3|4|5|6|7|8|9|10|11|12|13|14|15|16|17|18|19|20|21|22|23|24|25|26|27|28|29|30|31|32|33|34|35|36|37|38|39|40)
  Logical : xbsIndex_r4/Logical  logical_function=XNOR  inputs=2  en=off  latency=0  precision=User Defined  arith_type=Unsigned  n_bits=32  bin_pt=0  align_bp=on  dbl_ovrd=off  block_type=logical
      settings: xl_area=[31 0 0 31 0 0 0]  block_version=12.1
  Shift : xbsIndex_r4/Shift  shift_dir=Left  shift_bits=1  en=off  latency=0  precision=Full  arith_type=Unsigned  n_bits=7  bin_pt=0  quantization=Truncate  overflow=Wrap  dbl_ovrd=off  block_type=shift
      settings: xl_area=[0 0 0 0 0 0 0]  block_version=12.1
  Out1 : Outport
  wires:
  Constant0/1 -> Logical/2
  Delay_Line/1(Out2) -> Logical/1
  Logical/1 -> Corr/1(In1)
  Constant1/1 -> AddSub/2
  Corr/1(Out2) -> Shift/1
  Shift/1 -> AddSub/1
  In1/1 -> Delay_Line/1(In1)
  AddSub/1 -> Out1/1

== system receiver_overall_reset/Receiver/Sym-Chooser/2-10/Corr0 ==
  In1 : Inport
  AddSub : xbsIndex_r4/AddSub  mode=Subtraction  use_carryin=off  use_carryout=off  en=off  latency=0  precision=Full  arith_type=Unsigned  n_bits=16  bin_pt=14  quantization=Truncate  overflow=Wrap  dbl_ovrd=off  use_behavioral_HDL=off  hw_selection=Fabric  pipelined=off  block_type=addsub
      settings: xl_area=[4 0 0 6 0 0 0]  block_version=12.1
  Constant0 : xbsIndex_r4/Constant  arith_type=Unsigned  const=chip_a  n_bits=31  bin_pt=0  explicit_period=off  period=1/8  equ=P=C  opselect=C  inp2=PCIN>>17  opr=+  inp1=P  carry=CIN  dbl_ovrd=off  block_type=constant
      settings: block_version=12.1
  Constant1 : xbsIndex_r4/Constant  arith_type=Unsigned  const=31  n_bits=5  bin_pt=0  explicit_period=off  period=1/8  equ=P=C  opselect=C  inp2=PCIN>>17  opr=+  inp1=P  carry=CIN  dbl_ovrd=off  block_type=constant
      settings: block_version=12.1
  Corr : Subsystem
  Delay_Line : Subsystem  mask{bits=31}
      mask prompts: bits "Number of Bits [2-40]"
      mask init: same as receiver_overall_reset/Receiver/Sym-Clk/Corr/Delay_Line
      mask StyleString: popup(2|3|4|5|6|7|8|9|10|11|12|13|14|15|16|17|18|19|20|21|22|23|24|25|26|27|28|29|30|31|32|33|34|35|36|37|38|39|40)
  Logical : xbsIndex_r4/Logical  logical_function=XNOR  inputs=2  en=off  latency=0  precision=User Defined  arith_type=Unsigned  n_bits=32  bin_pt=0  align_bp=on  dbl_ovrd=off  block_type=logical
      settings: xl_area=[31 0 0 31 0 0 0]  block_version=12.1
  Shift : xbsIndex_r4/Shift  shift_dir=Left  shift_bits=1  en=off  latency=0  precision=Full  arith_type=Unsigned  n_bits=7  bin_pt=0  quantization=Truncate  overflow=Wrap  dbl_ovrd=off  block_type=shift
      settings: xl_area=[0 0 0 0 0 0 0]  block_version=12.1
  Out1 : Outport
  wires:
  Constant0/1 -> Logical/2
  Delay_Line/1(Out2) -> Logical/1
  Logical/1 -> Corr/1(In1)
  Constant1/1 -> AddSub/2
  Corr/1(Out2) -> Shift/1
  Shift/1 -> AddSub/1
  In1/1 -> Delay_Line/1(In1)
  AddSub/1 -> Out1/1

== system receiver_overall_reset/Receiver/Sym-Chooser/3-11/Corr0 ==
  In1 : Inport
  AddSub : xbsIndex_r4/AddSub  mode=Subtraction  use_carryin=off  use_carryout=off  en=off  latency=0  precision=Full  arith_type=Unsigned  n_bits=16  bin_pt=14  quantization=Truncate  overflow=Wrap  dbl_ovrd=off  use_behavioral_HDL=off  hw_selection=Fabric  pipelined=off  block_type=addsub
      settings: xl_area=[4 0 0 6 0 0 0]  block_version=12.1
  Constant0 : xbsIndex_r4/Constant  arith_type=Unsigned  const=chip_a  n_bits=31  bin_pt=0  explicit_period=off  period=1/8  equ=P=C  opselect=C  inp2=PCIN>>17  opr=+  inp1=P  carry=CIN  dbl_ovrd=off  block_type=constant
      settings: block_version=12.1
  Constant1 : xbsIndex_r4/Constant  arith_type=Unsigned  const=31  n_bits=5  bin_pt=0  explicit_period=off  period=1/8  equ=P=C  opselect=C  inp2=PCIN>>17  opr=+  inp1=P  carry=CIN  dbl_ovrd=off  block_type=constant
      settings: block_version=12.1
  Corr : Subsystem
  Delay_Line : Subsystem  mask{bits=31}
      mask prompts: bits "Number of Bits [2-40]"
      mask init: same as receiver_overall_reset/Receiver/Sym-Clk/Corr/Delay_Line
      mask StyleString: popup(2|3|4|5|6|7|8|9|10|11|12|13|14|15|16|17|18|19|20|21|22|23|24|25|26|27|28|29|30|31|32|33|34|35|36|37|38|39|40)
  Logical : xbsIndex_r4/Logical  logical_function=XNOR  inputs=2  en=off  latency=0  precision=User Defined  arith_type=Unsigned  n_bits=32  bin_pt=0  align_bp=on  dbl_ovrd=off  block_type=logical
      settings: xl_area=[31 0 0 31 0 0 0]  block_version=12.1
  Shift : xbsIndex_r4/Shift  shift_dir=Left  shift_bits=1  en=off  latency=0  precision=Full  arith_type=Unsigned  n_bits=7  bin_pt=0  quantization=Truncate  overflow=Wrap  dbl_ovrd=off  block_type=shift
      settings: xl_area=[0 0 0 0 0 0 0]  block_version=12.1
  Out1 : Outport
  wires:
  Constant0/1 -> Logical/2
  Delay_Line/1(Out2) -> Logical/1
  Logical/1 -> Corr/1(In1)
  Constant1/1 -> AddSub/2
  Corr/1(Out2) -> Shift/1
  Shift/1 -> AddSub/1
  In1/1 -> Delay_Line/1(In1)
  AddSub/1 -> Out1/1

== system receiver_overall_reset/Receiver/Sym-Chooser/4-12/Corr0 ==
  In1 : Inport
  AddSub : xbsIndex_r4/AddSub  mode=Subtraction  use_carryin=off  use_carryout=off  en=off  latency=0  precision=Full  arith_type=Unsigned  n_bits=16  bin_pt=14  quantization=Truncate  overflow=Wrap  dbl_ovrd=off  use_behavioral_HDL=off  hw_selection=Fabric  pipelined=off  block_type=addsub
      settings: xl_area=[4 0 0 6 0 0 0]  block_version=12.1
  Constant0 : xbsIndex_r4/Constant  arith_type=Unsigned  const=chip_a  n_bits=31  bin_pt=0  explicit_period=off  period=1/8  equ=P=C  opselect=C  inp2=PCIN>>17  opr=+  inp1=P  carry=CIN  dbl_ovrd=off  block_type=constant
      settings: block_version=12.1
  Constant1 : xbsIndex_r4/Constant  arith_type=Unsigned  const=31  n_bits=5  bin_pt=0  explicit_period=off  period=1/8  equ=P=C  opselect=C  inp2=PCIN>>17  opr=+  inp1=P  carry=CIN  dbl_ovrd=off  block_type=constant
      settings: block_version=12.1
  Corr : Subsystem
  Delay_Line : Subsystem  mask{bits=31}
      mask prompts: bits "Number of Bits [2-40]"
      mask init: same as receiver_overall_reset/Receiver/Sym-Clk/Corr/Delay_Line
      mask StyleString: popup(2|3|4|5|6|7|8|9|10|11|12|13|14|15|16|17|18|19|20|21|22|23|24|25|26|27|28|29|30|31|32|33|34|35|36|37|38|39|40)
  Logical : xbsIndex_r4/Logical  logical_function=XNOR  inputs=2  en=off  latency=0  precision=User Defined  arith_type=Unsigned  n_bits=32  bin_pt=0  align_bp=on  dbl_ovrd=off  block_type=logical
      settings: xl_area=[31 0 0 31 0 0 0]  block_version=12.1
  Shift : xbsIndex_r4/Shift  shift_dir=Left  shift_bits=1  en=off  latency=0  precision=Full  arith_type=Unsigned  n_bits=7  bin_pt=0  quantization=Truncate  overflow=Wrap  dbl_ovrd=off  block_type=shift
      settings: xl_area=[0 0 0 0 0 0 0]  block_version=12.1
  Out1 : Outport
  wires:
  Constant0/1 -> Logical/2
  Delay_Line/1(Out2) -> Logical/1
  Logical/1 -> Corr/1(In1)
  Constant1/1 -> AddSub/2
  Corr/1(Out2) -> Shift/1
  Shift/1 -> AddSub/1
  In1/1 -> Delay_Line/1(In1)
  AddSub/1 -> Out1/1

== system receiver_overall_reset/Receiver/Sym-Chooser/5-13/Corr0 ==
  In1 : Inport
  AddSub : xbsIndex_r4/AddSub  mode=Subtraction  use_carryin=off  use_carryout=off  en=off  latency=0  precision=Full  arith_type=Unsigned  n_bits=16  bin_pt=14  quantization=Truncate  overflow=Wrap  dbl_ovrd=off  use_behavioral_HDL=off  hw_selection=Fabric  pipelined=off  block_type=addsub
      settings: xl_area=[4 0 0 6 0 0 0]  block_version=12.1
  Constant0 : xbsIndex_r4/Constant  arith_type=Unsigned  const=chip_a  n_bits=31  bin_pt=0  explicit_period=off  period=1/8  equ=P=C  opselect=C  inp2=PCIN>>17  opr=+  inp1=P  carry=CIN  dbl_ovrd=off  block_type=constant
      settings: block_version=12.1
  Constant1 : xbsIndex_r4/Constant  arith_type=Unsigned  const=31  n_bits=5  bin_pt=0  explicit_period=off  period=1/8  equ=P=C  opselect=C  inp2=PCIN>>17  opr=+  inp1=P  carry=CIN  dbl_ovrd=off  block_type=constant
      settings: block_version=12.1
  Corr : Subsystem
  Delay_Line : Subsystem  mask{bits=31}
      mask prompts: bits "Number of Bits [2-40]"
      mask init: same as receiver_overall_reset/Receiver/Sym-Clk/Corr/Delay_Line
      mask StyleString: popup(2|3|4|5|6|7|8|9|10|11|12|13|14|15|16|17|18|19|20|21|22|23|24|25|26|27|28|29|30|31|32|33|34|35|36|37|38|39|40)
  Logical : xbsIndex_r4/Logical  logical_function=XNOR  inputs=2  en=off  latency=0  precision=User Defined  arith_type=Unsigned  n_bits=32  bin_pt=0  align_bp=on  dbl_ovrd=off  block_type=logical
      settings: xl_area=[31 0 0 31 0 0 0]  block_version=12.1
  Shift : xbsIndex_r4/Shift  shift_dir=Left  shift_bits=1  en=off  latency=0  precision=Full  arith_type=Unsigned  n_bits=7  bin_pt=0  quantization=Truncate  overflow=Wrap  dbl_ovrd=off  block_type=shift
      settings: xl_area=[0 0 0 0 0 0 0]  block_version=12.1
  Out1 : Outport
  wires:
  Constant0/1 -> Logical/2
  Delay_Line/1(Out2) -> Logical/1
  Logical/1 -> Corr/1(In1)
  Constant1/1 -> AddSub/2
  Corr/1(Out2) -> Shift/1
  Shift/1 -> AddSub/1
  In1/1 -> Delay_Line/1(In1)
  AddSub/1 -> Out1/1
